simulink model "INS"  (R2018b)
settings: configuration reference "ins_config" (kept outside this file)
values from neighbouring files (symbols this model uses):
  INS_EXPORT = Simulink.Parameter(INS_EXPORT_VALUE)    [ins_model_init.m]
  INS_PARAM = Simulink.Parameter(INS_PARAM_VALUE)    [ins_model_init.m]
undefined symbols (not defined in the file or in its folder): DiscIntNeverNeededParam, INS_CONST, INS_EXPORT_VALUE
libraries: simulink x90, FMT_Model_Lib x31
(part 2 of 4)

== system INS/Bus_Constructor/Status_Output/INS_Flag/valid_check8 ==
  quality : Inport
  Compare To Constant : simulink/Logic and Bit Operations/Compare To Constant  relop=>=  const=time_out  OutDataTypeStr=boolean
  Compare To Constant1 : simulink/Logic and Bit Operations/Compare To Constant  relop=>  const=0  OutDataTypeStr=boolean
  Compare To Constant2 : simulink/Logic and Bit Operations/Compare To Constant  relop=>  const=0  OutDataTypeStr=boolean
  Constant : Constant  Value=INS_EXPORT.period  OutDataTypeStr=Inherit: Inherit via back propagation
  Delay : Delay  DelayLength=1
  Detect Rise Positive : simulink/Logic and Bit Operations/Detect Rise Positive  vinit=0  OutDataTypeStr=boolean
  Discrete-Time Integrator : DiscreteIntegrator  IntegratorMethod=Accumulation: Forward Euler  gainval=1  ExternalReset=level  SampleTime=-1  LimitOutput=on  UpperSaturationLimit=1e6  LowerSaturationLimit=0  ICPrevOutput=DiscIntNeverNeededParam  ICPrevScaledInput=DiscIntNeverNeededParam
  Logical Operator : Logic  Operator=NOT  AllPortsSameDT=off  OutDataTypeStr=boolean
  Logical Operator1 : Logic  Operator=OR  AllPortsSameDT=off  OutDataTypeStr=boolean
  Multiply : Product
  valid : Outport
  wires:
  Multiply/1 -> valid/1
  Delay/1 -> Multiply/2, Logical Operator1/2
  Logical Operator1/1 -> Delay/1
  Detect Rise Positive/1 -> Logical Operator1/1
  Compare To Constant2/1 -> Detect Rise Positive/1
  quality/1 -> Compare To Constant1/1, Compare To Constant2/1
  Compare To Constant1/1 -> Discrete-Time Integrator/2
  Constant/1 -> Discrete-Time Integrator/1
  Discrete-Time Integrator/1 -> Compare To Constant/1
  Compare To Constant/1 -> Logical Operator/1
  Logical Operator/1 -> Multiply/1

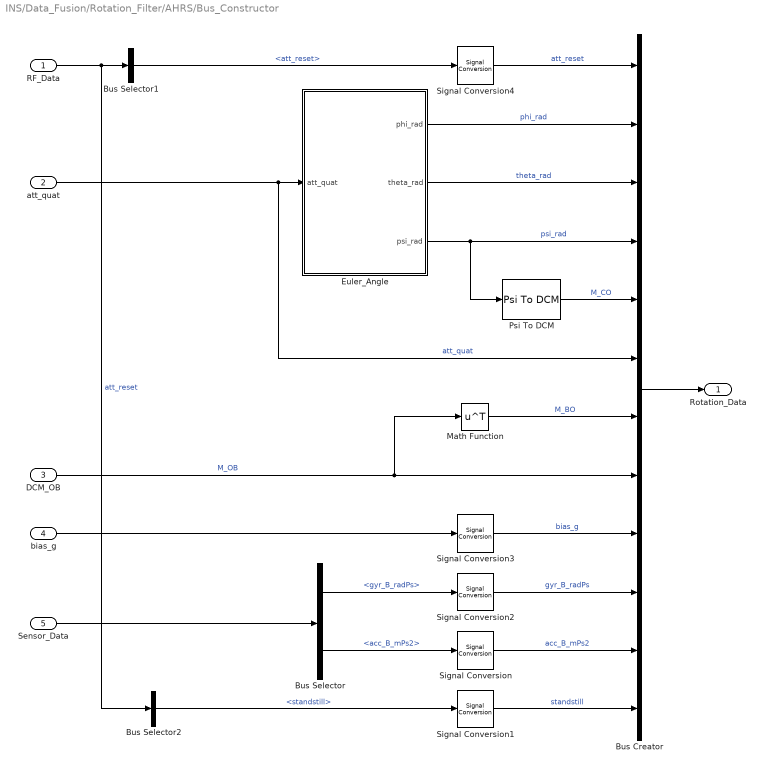
== system INS/Data_Fusion/Rotation_Filter/AHRS/Bus_Constructor ==
  RF_Data : Inport
  att_quat : Inport  Port=2
  DCM_OB : Inport  Port=3
  bias_g : Inport  Port=4
  Sensor_Data : Inport  Port=5
  Bus Creator : BusCreator  Inputs=12
  Bus Selector : BusSelector  OutputSignals=IMU_Data.gyr_B_radPs,IMU_Data.acc_B_mPs2
  Bus Selector1 : BusSelector  OutputSignals=att_reset
  Bus Selector2 : BusSelector  OutputSignals=standstill
  Euler_Angle : Subsystem
  Math Function : Math  Operator=transpose  SaturateOnIntegerOverflow=on
  Psi To DCM : FMT_Model_Lib/Transformation/Psi To DCM
      settings: SourceProductName=FMT Toolbox
  Signal Conversion{,1..4} (5 alike) : SignalConversion  OverrideOpt=off
  Rotation_Data : Outport
  wires:
  Bus Selector1/1 -> Signal Conversion4/1  "<att_reset>"
  Signal Conversion/1 -> Bus Creator/11  "acc_B_mPs2"
  Euler_Angle/1(phi_rad) -> Bus Creator/2  "phi_rad"
  Euler_Angle/2(theta_rad) -> Bus Creator/3  "theta_rad"
  Euler_Angle/3(psi_rad) -> Psi To DCM/1, Bus Creator/4  "psi_rad"
  Sensor_Data/1 -> Bus Selector/1
  Bus Selector2/1 -> Signal Conversion1/1  "<standstill>"
  Bus Creator/1 -> Rotation_Data/1
  bias_g/1 -> Signal Conversion3/1
  Math Function/1 -> Bus Creator/7  "M_BO"
  DCM_OB/1 -> Math Function/1, Bus Creator/8  "M_OB"
  att_quat/1 -> Euler_Angle/1(att_quat), Bus Creator/6  "att_quat"
  Psi To DCM/1 -> Bus Creator/5  "M_CO"
  Signal Conversion1/1 -> Bus Creator/12  "standstill"
  Bus Selector/2 -> Signal Conversion/1  "<acc_B_mPs2>"
  Signal Conversion2/1 -> Bus Creator/10  "gyr_B_radPs"
  Signal Conversion3/1 -> Bus Creator/9  "bias_g"
  RF_Data/1 -> Bus Selector2/1, Bus Selector1/1  "att_reset"
  Bus Selector/1 -> Signal Conversion2/1  "<gyr_B_radPs>"
  Signal Conversion4/1 -> Bus Creator/1  "att_reset"

== system INS/Data_Fusion/Rotation_Filter/AHRS/Correct ==
  Rotation_Data : Inport
  Sensor_Data : Inport  Port=2
  RF_Data : Inport  Port=3
  Attitude_Correction : Subsystem
  Bus Selector : BusSelector  OutputSignals=standstill
  Bus Selector1 : BusSelector  OutputSignals=IMU_Data
  Gyro_Bias_Correction : Subsystem
  att_B_correction : Outport
  bias_g_B_correction : Outport  Port=2
  wires:
  Gyro_Bias_Correction/1(bias_g_B_correction) -> bias_g_B_correction/1
  Bus Selector1/1 -> Gyro_Bias_Correction/2(IMU_Data)  "<IMU_Data>"
  RF_Data/1 -> Bus Selector/1
  Attitude_Correction/1(att_B_correction) -> att_B_correction/1, Gyro_Bias_Correction/1(att_B_correction)
  Sensor_Data/1 -> Attitude_Correction/1(Sensor_Data), Bus Selector1/1
  Rotation_Data/1 -> Attitude_Correction/2(Rotation_Data)
  Bus Selector/1 -> Attitude_Correction/3(standstill)  "<standstill>"

== system INS/Data_Fusion/Rotation_Filter/AHRS/Update ==
  att_B_correction : Inport
  bias_g_correction : Inport  Port=2
  RF_Data : Inport  Port=3
  Sensor_Data : Inport  Port=4
  Attitude_Update : Subsystem
  Bus Selector : BusSelector  OutputSignals=IMU_Data.gyr_B_radPs
  Bus Selector1 : BusSelector  OutputSignals=att_reset,quat_0
  Gyro_Bias_Update : Subsystem
  Sum2 : Sum  Inputs=|++
  att_quat : Outport
  DCM_OB : Outport  Port=2
  bias_g : Outport  Port=3
  wires:
  Sensor_Data/1 -> Bus Selector/1
  Gyro_Bias_Update/1(gyr_B_correction) -> Sum2/2
  att_B_correction/1 -> Sum2/1
  Sum2/1 -> Attitude_Update/3(att_B_correction)
  Bus Selector/1 -> Gyro_Bias_Update/2(gyr_B_radPs)  "<gyr_B_radPs>"
  bias_g_correction/1 -> Gyro_Bias_Update/1(bias_g_correction)
  Attitude_Update/1(att_quat) -> att_quat/1
  Attitude_Update/2(DCM_OB) -> DCM_OB/1
  Gyro_Bias_Update/2(bias_g) -> bias_g/1
  RF_Data/1 -> Bus Selector1/1  "att_reset"
  Bus Selector1/1 -> Attitude_Update/1(att_reset)  "<att_reset>"
  Bus Selector1/2 -> Attitude_Update/2(quat_0)  "<quat_0>"

== system INS/Data_Fusion/Rotation_Filter/RF_Data_PreProcess/Attitude_Reset ==
  Sensor_Data : Inport
  Bus Selector : BusSelector  OutputSignals=IMU_Data.IMU_valid,Mag_Data.mag_quality,IMU_Data.acc_B_mPs2,Mag_Data.mag_norm_B
  Bus Selector1 : BusSelector  OutputSignals=GPS_Data.GPS_valid
  Compare To Constant : simulink/Logic and Bit Operations/Compare To Constant  relop=>  const=0.01  OutDataTypeStr=boolean
  Compare To Constant1 : simulink/Logic and Bit Operations/Compare To Constant  relop=>=  const=0.2  OutDataTypeStr=boolean
  Detect Rise Positive : simulink/Logic and Bit Operations/Detect Rise Positive  vinit=0  OutDataTypeStr=boolean
  Interval Test : simulink/Logic and Bit Operations/Interval Test  IntervalClosedRight=on  uplimit=INS_CONST.g+0.5  IntervalClosedLeft=on  lowlimit=INS_CONST.g-0.5  OutDataTypeStr=boolean
  Logical Operator : Logic  AllPortsSameDT=off  OutDataTypeStr=boolean
  Logical Operator1 : Logic  Inputs=4  AllPortsSameDT=off  OutDataTypeStr=boolean
  Logical Operator2 : Logic  Operator=OR  AllPortsSameDT=off  OutDataTypeStr=boolean
  Reset Heading : Subsystem
  Vector Modulus : FMT_Model_Lib/Math/Vector Modulus
      settings: SourceProductName=FMT Toolbox
  Vector Modulus1 : FMT_Model_Lib/Math/Vector Modulus
      settings: SourceProductName=FMT Toolbox
  sample_valid : Subsystem
  att_reset : Outport
  wires:
  sample_valid/1(sample_valid) -> Logical Operator/1, Detect Rise Positive/1
  Vector Modulus1/1 -> Compare To Constant/1
  Compare To Constant/1 -> Logical Operator1/4
  Interval Test/1 -> Logical Operator1/3
  Vector Modulus/1 -> Interval Test/1
  Logical Operator1/1 -> sample_valid/1(valid)
  Sensor_Data/1 -> Bus Selector1/1, Bus Selector/1
  Bus Selector/2 -> Compare To Constant1/1  "<mag_quality>"
  Bus Selector/3 -> Vector Modulus/1  "<acc_B_mPs2>"
  Bus Selector/1 -> Logical Operator1/1  "<IMU_valid>"
  Compare To Constant1/1 -> Logical Operator1/2
  Bus Selector/4 -> Vector Modulus1/1  "<mag_norm_B>"
  Detect Rise Positive/1 -> Logical Operator2/1
  Logical Operator/1 -> Logical Operator2/2
  Logical Operator2/1 -> att_reset/1
  Bus Selector1/1 -> Reset Heading/1(GPS_valid)  "<GPS_valid>"
  Reset Heading/1(reset) -> Logical Operator/2

== system INS/Data_Fusion/Rotation_Filter/RF_Data_PreProcess/Initial_Attitude ==
  Sensor_Data : Inport
  Enable : EnablePort
  Bus Selector : BusSelector  OutputSignals=IMU_Data.acc_B_mPs2,Mag_Data.mag_norm_B
  Cross Product : FMT_Model_Lib/Math/Cross Product
      settings: SourceProductName=FMT Toolbox
  Cross Product1 : FMT_Model_Lib/Math/Cross Product
      settings: SourceProductName=FMT Toolbox
  DCM To Quaternion : FMT_Model_Lib/Quaternion/DCM To Quaternion
      settings: SourceProductName=FMT Toolbox
  Gain : Gain  Gain=-1
  Vector Concatenate : Concatenate  NumInputs=3  Mode=Multidimensional array  ConcatenateDimension=2
  Vector Normalize : FMT_Model_Lib/Math/Vector Normalize
      settings: SourceProductName=FMT Toolbox
  Vector Normalize1 : FMT_Model_Lib/Math/Vector Normalize
      settings: SourceProductName=FMT Toolbox
  Vector Normalize2 : FMT_Model_Lib/Math/Vector Normalize
      settings: SourceProductName=FMT Toolbox
  quat_0 : Outport  InitialOutput=[1; 0; 0; 0]
  wires:
  Gain/1 -> Cross Product/1, Vector Normalize2/1, Cross Product1/2
  Cross Product1/1 -> Vector Normalize/1
  Cross Product/1 -> Vector Normalize1/1, Cross Product1/1
  Vector Normalize1/1 -> Vector Concatenate/2  "DCM_y"
  Vector Normalize/1 -> Vector Concatenate/1  "DCM_x"
  Vector Normalize2/1 -> Vector Concatenate/3  "DCM_z"
  DCM To Quaternion/1 -> quat_0/1
  Sensor_Data/1 -> Bus Selector/1
  Bus Selector/1 -> Gain/1  "<acc_B_mPs2>"
  Bus Selector/2 -> Cross Product/2  "<mag_norm_B>"
  Vector Concatenate/1 -> DCM To Quaternion/1  "M_BO"

== system INS/Data_Fusion/Rotation_Filter/RF_Data_PreProcess/Standstill ==
  IMU_Data : Inport
  Abs : Abs
  Bus Selector : BusSelector  OutputSignals=gyr_B_radPs
  First Order HPF : FMT_Model_Lib/Filter/First Order HPF  fc=1/(2*pi*0.25)
      settings: SourceProductName=FMT Toolbox
  First Order LPF : FMT_Model_Lib/Filter/First Order LPF  fc=1/(2*pi*0.5)
      settings: SourceProductName=FMT Toolbox
  First Order LPF1 : FMT_Model_Lib/Filter/First Order LPF  fc=1/(2*pi*0.05)
      settings: SourceProductName=FMT Toolbox
  MinMax1 : MinMax  Function=max
  Relay : Relay  OnSwitchValue=10e-3  OffSwitchValue=3e-3  OnOutputValue=0  OffOutputValue=1
  Saturation2 : Saturate  UpperLimit=1  LowerLimit=0
  Selector : Selector  InputPortWidth=3  IndexOptions=Index vector (dialog)  Indices=[1 2]  OutputSizes=1
  standstill : Outport
  wires:
  First Order LPF1/1 -> Relay/1
  Relay/1 -> standstill/1
  Saturation2/1 -> First Order LPF1/1
  First Order HPF/1 -> Abs/1
  Selector/1 -> First Order HPF/1
  Abs/1 -> MinMax1/1
  First Order LPF/1 -> Saturation2/1
  MinMax1/1 -> First Order LPF/1
  Bus Selector/1 -> Selector/1  "<gyr_B_radPs>"
  IMU_Data/1 -> Bus Selector/1

== system INS/Data_Fusion/Translation_Filter/CF/Bus_Constructor ==
  TF_Data : Inport
  Horizontal_States : Inport  Port=2
  Verticle_States : Inport  Port=3
  Bus Creator : BusCreator  Inputs=16
  Bus Selector : BusSelector  OutputSignals=Sensor_Enable,TF_Control.WGS84_Ref.WGS84_pos_ref.lat_0_rad,TF_Control.WGS84_Ref.WGS84_pos_ref.lon_0_rad,TF_Control.WGS84_Ref.WGS84_pos_ref.h_0_m
  Bus_Select : Subsystem
  Constant : Constant  OutDataTypeStr=Inherit: Inherit via back propagation
  Signal Copy{,1..3} (4 alike) : SignalConversion  OverrideOpt=off
  Translation_Data : Outport
  wires:
  Bus Creator/1 -> Translation_Data/1
  Bus_Select/10(vd_mPs) -> Bus Creator/10  "vd_mPs"
  Bus_Select/9(ve_mPs) -> Bus Creator/9  "ve_mPs"
  Bus_Select/8(vn_mPs) -> Bus Creator/8  "vn_mPs"
  Bus_Select/3(h_m) -> Bus Creator/3  "h_m"
  Bus_Select/2(lon_rad) -> Bus Creator/2  "lon_rad"
  Bus_Select/1(lat_rad) -> Bus Creator/1  "lat_rad"
  Bus_Select/11(ba_mPs2) -> Bus Creator/11  "ba_mPs2"
  Verticle_States/1 -> Bus_Select/2(Verticle_States)
  Horizontal_States/1 -> Bus_Select/1(Horizontal_States)
  TF_Data/1 -> Bus Selector/1, Bus_Select/3(TF_Data)
  Constant/1 -> Bus Creator/16  "init_done"
  Bus_Select/7(h_gnd_m) -> Bus Creator/7  "h_gnd_m"
  Bus_Select/6(h_R_m) -> Bus Creator/6  "h_R_m"
  Bus_Select/4(x_R_m) -> Bus Creator/4  "x_R_m"
  Bus_Select/5(y_R_m) -> Bus Creator/5  "y_R_m"
  Bus Selector/1 -> Signal Copy/1  "<Sensor_Enable>"
  Signal Copy/1 -> Bus Creator/12  "sensor_enable"
  Bus Selector/2 -> Signal Copy1/1  "<lat_0_rad>"
  Bus Selector/3 -> Signal Copy2/1  "<lon_0_rad>"
  Bus Selector/4 -> Signal Copy3/1  "<h_0_m>"
  Signal Copy1/1 -> Bus Creator/13  "lat_0_rad"
  Signal Copy2/1 -> Bus Creator/14  "lon_0_rad"
  Signal Copy3/1 -> Bus Creator/15  "h_0_m"

== system INS/Data_Fusion/Translation_Filter/CF/Horizontal_Filter ==
  TF_Data : Inport
  Rotation_Data : Inport  Port=2
  Correct : Subsystem
  Predict : Subsystem
  Reshape : Reshape  OutputDimensionality=Customize  OutputDimensions=[6,1]
  States : Outport
  wires:
  Predict/1(X_Predict) -> Correct/1(X_Predict)
  Correct/1(X_Next) -> Reshape/1
  Reshape/1 -> Predict/1(X_Prio), States/1
  TF_Data/1 -> Correct/2(TF_Data), Predict/3(TF_Data)
  Rotation_Data/1 -> Predict/2(Rotation_Data)

== system INS/Data_Fusion/Translation_Filter/CF/Verticle_Filter ==
  TF_Data : Inport
  Rotation_Data : Inport  Port=2
  Correct : Subsystem
  Predict : Subsystem
  Reshape : Reshape  OutputDimensionality=Customize  OutputDimensions=[3,1]
  States : Outport
  wires:
  Predict/1(X_Predict) -> Correct/1(X_Predict)
  Correct/1(X_Next) -> Reshape/1
  Reshape/1 -> Predict/1(X_Prio), States/1
  TF_Data/1 -> Correct/2(TF_Data), Predict/3(TF_Data)
  Rotation_Data/1 -> Predict/2(Rotation_Data)

== system INS/Data_Fusion/Translation_Filter/TF_Data_PreProcess/Sensor_Process ==
  Sensor_Data : Inport
  Sensor_Select : Subsystem
  TF_Sensor_Measures : Subsystem
  TF_Sensor_Status : Subsystem
  Sensor_Status : Outport
  Sensor_Meas : Outport  Port=2
  Sensor_Enable : Outport  Port=3
  wires:
  Sensor_Data/1 -> TF_Sensor_Measures/1(Sensor_Data), TF_Sensor_Status/1(Sensor_Data)
  TF_Sensor_Measures/1(Sensor_Meas) -> Sensor_Meas/1
  TF_Sensor_Status/1(Sensor_Status) -> Sensor_Select/1(Sensor_Status), Sensor_Status/1
  Sensor_Select/1(Sensor_Select) -> Sensor_Enable/1  "Sensor_Enable"

== system INS/Data_Fusion/Translation_Filter/TF_Data_PreProcess/Transfer_Filter_Control ==
  Sensor_Enable : Inport
  Sensor_Meas : Inport  Port=2
  Translation_Data : Inport  Port=3
  Bus Creator : BusCreator  Inputs=4
  Filter_Reset : Subsystem
  Position_Reference : Subsystem
  Sensor_Valid : Subsystem
  TF_Control : Outport
  wires:
  Position_Reference/1(WGS84_Ref) -> Bus Creator/4  "WGS84_Ref"
  Sensor_Meas/1 -> Position_Reference/3(Sensor_Meas)
  Filter_Reset/1(pos_reset) -> Bus Creator/1  "pos_reset"
  Sensor_Enable/1 -> Sensor_Valid/1(Sensor_Enable)
  Filter_Reset/2(height_reset) -> Bus Creator/2  "height_reset"
  Bus Creator/1 -> TF_Control/1
  Translation_Data/1 -> Position_Reference/2(Translation_Data)
  Sensor_Valid/1(Sensor_Valid) -> Position_Reference/1(Sensor_Valid), Bus Creator/3, Filter_Reset/1(Sensor_Valid)  "sensor_valid"

== system INS/Sensor_PreProcess/Baro_Process/Relative_Height/Reference_Height ==
  h_FL_m : Inport
  Enable : EnablePort  StatesWhenEnabling=reset
  Constant1 : Constant  OutDataTypeStr=uint32
  Delay : Delay  DelayLength=1
  Delay1 : Delay  DelayLength=1
  Divide : Product  Inputs=*/
  Saturation1 : Saturate  UpperLimit=10000  LowerLimit=1
  Sum1 : Sum  Inputs=|++  AccumDataTypeStr=uint32  OutDataTypeStr=uint32  RndMeth=Simplest  SaturateOnIntegerOverflow=on
  Sum2 : Sum  Inputs=|++
  h_R_m : Outport
  wires:
  Saturation1/1 -> Divide/2
  Constant1/1 -> Sum1/1
  Sum1/1 -> Delay1/1, Saturation1/1
  Delay1/1 -> Sum1/2
  Sum2/1 -> Delay/1, Divide/1
  Delay/1 -> Sum2/2
  h_FL_m/1 -> Sum2/1
  Divide/1 -> h_R_m/1

== system INS/Sensor_PreProcess/Baro_Process/Relative_Height/Sampling ==
  timestamp : Inport
  data_valid : Inport  Port=2
  Compare To Constant : simulink/Logic and Bit Operations/Compare To Constant  relop=>  const=200  OutDataTypeStr=boolean
  Delay : Delay  DelayLength=1
  Detect Change : simulink/Logic and Bit Operations/Detect Change  vinit=0  OutDataTypeStr=boolean
  Interval Test3 : simulink/Logic and Bit Operations/Interval Test  IntervalClosedRight=off  uplimit=200  IntervalClosedLeft=off  lowlimit=1  OutDataTypeStr=boolean
  Logical Operator5 : Logic  AllPortsSameDT=off  OutDataTypeStr=boolean
  Saturation : Saturate  UpperLimit=10000  LowerLimit=0
  Sum1 : Sum  Inputs=|++  AccumDataTypeStr=uint32  OutDataTypeStr=uint32  RndMeth=Simplest  SaturateOnIntegerOverflow=on
  sampling : Outport
  initialized : Outport  Port=2
  wires:
  Detect Change/1 -> Logical Operator5/1
  Interval Test3/1 -> sampling/1
  Logical Operator5/1 -> Sum1/1
  Delay/1 -> Saturation/1
  timestamp/1 -> Detect Change/1
  data_valid/1 -> Logical Operator5/2
  Sum1/1 -> Interval Test3/1, Compare To Constant/1, Delay/1
  Saturation/1 -> Sum1/2
  Compare To Constant/1 -> initialized/1

== system INS/Sensor_PreProcess/GPS_PreProcess/Status_Quality/GPS_Status ==
  note: GPS Status
      | 0: Idle
      | 1: Ready, 3D fix lost
      | 2: Ready, 3D fix
  not_timeout : Inport
  hAcc : Inport  Port=2
  fixtype : Inport  Port=3
  Compare To Constant : simulink/Logic and Bit Operations/Compare To Constant  relop=<  const=5*1e3  OutDataTypeStr=uint8
  Compare To Constant1 : simulink/Logic and Bit Operations/Compare To Constant  relop===  const=3  OutDataTypeStr=uint8
  Logical Operator : Logic  Inputs=3  AllPortsSameDT=off  OutDataTypeStr=fixdt(0,8)
  Logical Operator1 : Logic  Inputs=3  AllPortsSameDT=off  OutDataTypeStr=fixdt(0,8)
  Ready : Subsystem
  Sum1 : Sum  Inputs=|++
  status : Outport
  wires:
  not_timeout/1 -> Logical Operator/3, Logical Operator1/3
  Sum1/1 -> status/1
  Logical Operator1/1 -> Sum1/2  "3D Fix"
  hAcc/1 -> Compare To Constant/1
  Compare To Constant/1 -> Logical Operator/1
  Compare To Constant1/1 -> Logical Operator1/2, Logical Operator/2  "3D Fix"
  fixtype/1 -> Compare To Constant1/1
  Ready/1(ready) -> Sum1/1, Logical Operator1/1  "ready"
  Logical Operator/1 -> Ready/1(valid)

== system INS/Sensor_PreProcess/GPS_PreProcess/Status_Quality/check_timeout ==
  timestamp : Inport
  Compare To Constant4 : simulink/Logic and Bit Operations/Compare To Constant  relop=<  const=500  OutDataTypeStr=boolean
  Constant : Constant  Value=INS_EXPORT.period  OutDataTypeStr=single
  Detect Change : simulink/Logic and Bit Operations/Detect Change  vinit=0  OutDataTypeStr=boolean
  Discrete-Time Integrator : DiscreteIntegrator  IntegratorMethod=Accumulation: Forward Euler  ExternalReset=sampled level  SampleTime=-1  OutDataTypeStr=uint32  SaturateOnIntegerOverflow=on  UpperSaturationLimit=10000  LowerSaturationLimit=0  ICPrevOutput=DiscIntNeverNeededParam  ICPrevScaledInput=DiscIntNeverNeededParam
  valid : Outport
  wires:
  Constant/1 -> Discrete-Time Integrator/1
  timestamp/1 -> Detect Change/1
  Detect Change/1 -> Discrete-Time Integrator/2
  Discrete-Time Integrator/1 -> Compare To Constant4/1
  Compare To Constant4/1 -> valid/1

== system INS/Sensor_PreProcess/GPS_PreProcess/Status_Quality/horizontal_quality ==
  hAcc : Inport
  Constant1 : Constant  Value=INS_PARAM.GPS_HOR_Q_BIAS  OutDataTypeStr=Inherit: Inherit via back propagation
  Gain1 : Gain  Gain=1e-3  OutDataTypeStr=single
  Gain2 : Gain  Gain=INS_PARAM.GPS_HOR_Q_SCALE  OutDataTypeStr=single
  Saturation1 : Saturate  UpperLimit=1  LowerLimit=0
  Sum1 : Sum  Inputs=+-|
  hor_quality : Outport
  wires:
  Sum1/1 -> Gain2/1
  Gain1/1 -> Sum1/2  "hAcc_m"
  hAcc/1 -> Gain1/1
  Constant1/1 -> Sum1/1
  Gain2/1 -> Saturation1/1
  Saturation1/1 -> hor_quality/1

== system INS/Sensor_PreProcess/GPS_PreProcess/Status_Quality/speed_acc ==
  sAcc : Inport
  Constant7 : Constant  Value=INS_PARAM.GPS_VEL_Q_BIAS  OutDataTypeStr=Inherit: Inherit via back propagation
  Gain3 : Gain  Gain=INS_PARAM.GPS_VEL_Q_SCALE  OutDataTypeStr=single
  Gain5 : Gain  Gain=1e-3  OutDataTypeStr=single
  Saturation : Saturate  UpperLimit=1  LowerLimit=0
  Second Order LPF : FMT_Model_Lib/Filter/Second Order LPF  fc=5  zeta=0.707
      settings: SourceProductName=FMT Toolbox
  Sum : Sum  Inputs=+-|
  spd_quality : Outport
  wires:
  Gain5/1 -> Sum/2  "sAcc_m"
  Sum/1 -> Gain3/1
  sAcc/1 -> Gain5/1
  Constant7/1 -> Sum/1
  Saturation/1 -> spd_quality/1
  Gain3/1 -> Second Order LPF/1
  Second Order LPF/1 -> Saturation/1

== system INS/Sensor_PreProcess/GPS_PreProcess/Status_Quality/vertical_quality ==
  vAcc : Inport
  Constant1 : Constant  Value=INS_PARAM.GPS_VER_Q_BIAS  OutDataTypeStr=Inherit: Inherit via back propagation
  Gain1 : Gain  Gain=1e-3  OutDataTypeStr=single
  Gain2 : Gain  Gain=INS_PARAM.GPS_VER_Q_SCALE  OutDataTypeStr=single
  Saturation1 : Saturate  UpperLimit=1  LowerLimit=0
  Sum1 : Sum  Inputs=+-|
  ver_quality : Outport
  wires:
  Sum1/1 -> Gain2/1
  Gain1/1 -> Sum1/2  "vAcc_m"
  vAcc/1 -> Gain1/1
  Constant1/1 -> Sum1/1
  Gain2/1 -> Saturation1/1
  Saturation1/1 -> ver_quality/1

== system INS/Sensor_PreProcess/MAG_PreProcess/Mag_Data_Process/Mag_Quality_Estimate ==
  note: TODO: improve this
  mag_normalized_O : Inport
  nominal_inc_deg : Inport  Port=2
  pos_0_valid : Inport  Port=3
  mag_valid : Inport  Port=4
  Mag_Quality : Subsystem
  Multiply : Product  OutDataTypeStr=Inherit: Same as first input
  Switch : Switch  Criteria=u2 > Threshold
  default_mag_quality : Constant  Value=0.5  OutDataTypeStr=single
  mag_quality : Outport
  wires:
  pos_0_valid/1 -> Switch/2
  default_mag_quality/1 -> Switch/3
  mag_valid/1 -> Multiply/2
  Switch/1 -> Multiply/1
  Multiply/1 -> mag_quality/1
  nominal_inc_deg/1 -> Mag_Quality/1(nominal_inc_deg)
  mag_normalized_O/1 -> Mag_Quality/2(mag_normalized_O)
  Mag_Quality/1(mag_quality) -> Switch/1

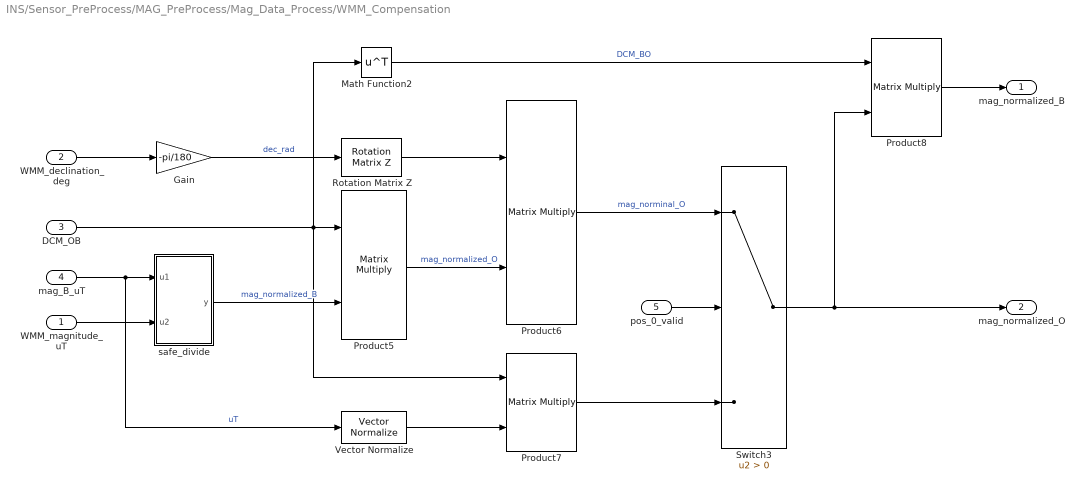
== system INS/Sensor_PreProcess/MAG_PreProcess/Mag_Data_Process/WMM_Compensation ==
  WMM_magnitude_uT : Inport
  WMM_declination_deg : Inport  Port=2
  DCM_OB : Inport  Port=3
  mag_B_uT : Inport  Port=4
  pos_0_valid : Inport  Port=5
  Gain : Gain  Gain=-pi/180  OutDataTypeStr=single
  Math Function2 : Math  Operator=transpose  SaturateOnIntegerOverflow=on
  Product{5..8} (4 alike) : Product  Multiplication=Matrix(*)
  Rotation Matrix Z : FMT_Model_Lib/Transformation/Rotation Matrix Z
      settings: SourceProductName=FMT Toolbox
  Switch3 : Switch  Criteria=u2 > Threshold
  Vector Normalize : FMT_Model_Lib/Math/Vector Normalize
      settings: SourceProductName=FMT Toolbox
  safe_divide : Subsystem
      mask Display:
      | port_label('input', 1, 'x', 'texmode', 'on')
      | port_label('input', 2, '÷', 'texmode', 'on')
  mag_normalized_B : Outport
  mag_normalized_O : Outport  Port=2
  wires:
  Gain/1 -> Rotation Matrix Z/1  "dec_rad"
  WMM_declination_deg/1 -> Gain/1
  mag_B_uT/1 -> Vector Normalize/1, safe_divide/1(u1)  "uT"
  WMM_magnitude_uT/1 -> safe_divide/2(u2)
  safe_divide/1(y) -> Product5/2  "mag_normalized_B"
  DCM_OB/1 -> Product5/1, Math Function2/1, Product7/1
  Product5/1 -> Product6/2  "mag_normalized_O"
  Rotation Matrix Z/1 -> Product6/1
  Product6/1 -> Switch3/1  "mag_norminal_O"
  Math Function2/1 -> Product8/1  "DCM_BO"
  pos_0_valid/1 -> Switch3/2
  Product8/1 -> mag_normalized_B/1
  Switch3/1 -> mag_normalized_O/1, Product8/2
  Vector Normalize/1 -> Product7/2
  Product7/1 -> Switch3/3

== system INS/Sensor_PreProcess/MAG_PreProcess/Mag_Data_Process/WMM_LUT ==
  lat_rad : Inport
  lon_rad : Inport  Port=2
  Add : Sum
  Declination_Lookup_Table : LookupNDDirect  Table=wmm_declination  DiagnosticForOutOfRangeInput=Error
  Demux : Demux  Outputs=2
  Inclination_Lookup_Table : LookupNDDirect  Table=wmm_inclination  DiagnosticForOutOfRangeInput=Error
  Magnitude_Lookup_Table : LookupNDDirect  Table=wmm_magnitude  DiagnosticForOutOfRangeInput=Error
  Mux : Mux  Inputs=2
  Saturation1 : Saturate  UpperLimit=size(wmm_magnitude)-1  LowerLimit=0
  offset : Constant  Value=(size(wmm_magnitude)-1)/2  OutDataTypeStr=int32
  rad_to_index : Gain  Gain=180/pi/resolution  OutDataTypeStr=int32
  magnitude_uT : Outport
  declination_deg : Outport  Port=2
  inclination_deg : Outport  Port=3
  wires:
  Inclination_Lookup_Table/1 -> inclination_deg/1
  Declination_Lookup_Table/1 -> declination_deg/1
  Magnitude_Lookup_Table/1 -> magnitude_uT/1
  offset/1 -> Add/2
  Add/1 -> Saturation1/1
  rad_to_index/1 -> Add/1
  lat_rad/1 -> Mux/1
  lon_rad/1 -> Mux/2
  Mux/1 -> rad_to_index/1
  Saturation1/1 -> Demux/1
  Demux/1 -> Magnitude_Lookup_Table/1, Inclination_Lookup_Table/1, Declination_Lookup_Table/1
  Demux/2 -> Inclination_Lookup_Table/2, Magnitude_Lookup_Table/2, Declination_Lookup_Table/2

== system INS/Data_Fusion/Rotation_Filter/AHRS/Bus_Constructor/Euler_Angle ==
  att_quat : Inport
  Demux : Demux  Outputs=3
  Quaternion To Euler : FMT_Model_Lib/Quaternion/Quaternion To Euler
      settings: SourceProductName=FMT Toolbox
  phi_rad : Outport
  theta_rad : Outport  Port=2
  psi_rad : Outport  Port=3
  wires:
  Demux/1 -> phi_rad/1
  Demux/2 -> theta_rad/1
  Demux/3 -> psi_rad/1
  att_quat/1 -> Quaternion To Euler/1
  Quaternion To Euler/1 -> Demux/1

== system INS/Data_Fusion/Rotation_Filter/AHRS/Correct/Attitude_Correction ==
  Sensor_Data : Inport
  Rotation_Data : Inport  Port=2
  standstill : Inport  Port=3
  Attitude_Correct : Subsystem
  Bus Selector2 : BusSelector  OutputSignals=M_BO
  Mag_Correct : Subsystem
  Multiply : Product  Multiplication=Matrix(*)
  Sum : Sum  Inputs=|++
  att_B_correction : Outport
  wires:
  standstill/1 -> Mag_Correct/3(standstill)
  Sensor_Data/1 -> Attitude_Correct/2(Sensor_Data), Mag_Correct/2(Sensor_Data)
  Attitude_Correct/1(att_corr_O) -> Sum/1  "att_corr_O"
  Mag_Correct/1(mag_corr_O) -> Sum/2  "mag_corr_O"
  Multiply/1 -> att_B_correction/1
  Rotation_Data/1 -> Mag_Correct/1(Rotation_Data), Attitude_Correct/1(Rotation_Data), Bus Selector2/1
  Sum/1 -> Multiply/2
  Bus Selector2/1 -> Multiply/1  "<M_BO>"

== system INS/Data_Fusion/Rotation_Filter/AHRS/Correct/Gyro_Bias_Correction ==
  att_B_correction : Inport
  IMU_Data : Inport  Port=2
  Abs : Abs
  Bus Selector : BusSelector  OutputSignals=acc_B_mPs2
  Compare To Constant : simulink/Logic and Bit Operations/Compare To Constant  relop=<=  const=1  OutDataTypeStr=boolean
  Constant : Constant  Value=INS_CONST.g  OutDataTypeStr=single
  Data Type Conversion : DataTypeConversion  OutDataTypeStr=single
  Gain1 : Gain  Gain=INS_PARAM.BIAS_G_CORR_GAIN
  MX Product1 : Product  RndMeth=Simplest
  Saturation2 : Saturate  UpperLimit=0.1/180*pi  LowerLimit=-0.1/180*pi
  Second Order LPF : FMT_Model_Lib/Filter/Second Order LPF  fc=5  zeta=0.707
      settings: SourceProductName=FMT Toolbox
  Subtract : Sum  Inputs=+-
  Vector Modulus : FMT_Model_Lib/Math/Vector Modulus
      settings: SourceProductName=FMT Toolbox
  bias_g_B_correction : Outport
  wires:
  IMU_Data/1 -> Bus Selector/1
  Saturation2/1 -> bias_g_B_correction/1  "bias_g_correction"
  Compare To Constant/1 -> Data Type Conversion/1
  Bus Selector/1 -> Vector Modulus/1  "<acc_B_mPs2>"
  MX Product1/1 -> Second Order LPF/1
  att_B_correction/1 -> MX Product1/1
  Vector Modulus/1 -> Subtract/1
  Gain1/1 -> Saturation2/1
  Constant/1 -> Subtract/2
  Subtract/1 -> Abs/1
  Abs/1 -> Compare To Constant/1
  Data Type Conversion/1 -> MX Product1/2
  Second Order LPF/1 -> Gain1/1

== system INS/Data_Fusion/Rotation_Filter/AHRS/Update/Attitude_Update ==
  att_reset : Inport
  quat_0 : Inport  Port=2
  att_B_correction : Inport  Port=3
  Constant : Constant  Value=0  OutDataTypeStr=single
  Discrete-Time Integrator : DiscreteIntegrator  ExternalReset=level  InitialConditionSource=external  SampleTime=-1  ICPrevOutput=DiscIntNeverNeededParam  ICPrevScaledInput=DiscIntNeverNeededParam
  Gain2 : Gain  Gain=0.5  OutMin=-450*pi/180  OutMax=450*pi/180  RndMeth=Simplest
  Mux1 : Mux  Inputs=2
  Quaternion Multiply : FMT_Model_Lib/Quaternion/Quaternion Multiply
      settings: SourceProductName=FMT Toolbox
  Quaternion Normalize : FMT_Model_Lib/Quaternion/Quaternion Normalize
      settings: SourceProductName=FMT Toolbox
  Quaternion To DCM : FMT_Model_Lib/Quaternion/Quaternion To DCM
      settings: SourceProductName=FMT Toolbox
  Transpose : Math  Operator=transpose  SaturateOnIntegerOverflow=on
  att_quat : Outport
  DCM_OB : Outport  Port=2
  wires:
  att_reset/1 -> Discrete-Time Integrator/2
  quat_0/1 -> Discrete-Time Integrator/3
  Gain2/1 -> Discrete-Time Integrator/1
  Quaternion Multiply/1 -> Gain2/1
  att_B_correction/1 -> Mux1/2
  Mux1/1 -> Quaternion Multiply/2
  Constant/1 -> Mux1/1
  Quaternion Normalize/1 -> Quaternion To DCM/1, Quaternion Multiply/1, att_quat/1
  Discrete-Time Integrator/1 -> Quaternion Normalize/1
  Quaternion To DCM/1 -> Transpose/1
  Transpose/1 -> DCM_OB/1

== system INS/Data_Fusion/Rotation_Filter/AHRS/Update/Gyro_Bias_Update ==
  bias_g_correction : Inport
  gyr_B_radPs : Inport  Port=2
  Discrete-Time Integrator2 : DiscreteIntegrator  SampleTime=-1  LimitOutput=on  UpperSaturationLimit=45/180*pi  LowerSaturationLimit=-45/180*pi  ICPrevOutput=DiscIntNeverNeededParam  ICPrevScaledInput=DiscIntNeverNeededParam
  Sum1 : Sum  Inputs=++|
  gyr_B_correction : Outport
  bias_g : Outport  Port=2
  wires:
  bias_g_correction/1 -> Discrete-Time Integrator2/1
  Sum1/1 -> gyr_B_correction/1
  Discrete-Time Integrator2/1 -> Sum1/1, bias_g/1
  gyr_B_radPs/1 -> Sum1/2

== system INS/Data_Fusion/Rotation_Filter/RF_Data_PreProcess/Attitude_Reset/Reset Heading ==
  note: When GPS is valid at first time, the mag data will be compensated with WMM data,
      | so we need reset attitude.
  GPS_valid : Inport
  Add : Sum  AccumDataTypeStr=uint32
  Data Type Conversion : DataTypeConversion  OutDataTypeStr=uint32
  Delay : Delay  DelayLength=1
  Detect Rise Positive1 : simulink/Logic and Bit Operations/Detect Rise Positive  vinit=0  OutDataTypeStr=boolean
  Saturation : Saturate  UpperLimit=1  LowerLimit=0
  reset : Outport
  wires:
  Delay/1 -> Add/2
  Data Type Conversion/1 -> Add/1
  GPS_valid/1 -> Data Type Conversion/1
  Detect Rise Positive1/1 -> reset/1
  Add/1 -> Saturation/1
  Saturation/1 -> Detect Rise Positive1/1, Delay/1

== system INS/Data_Fusion/Rotation_Filter/RF_Data_PreProcess/Attitude_Reset/sample_valid ==
  valid : Inport
  Add : Sum  AccumDataTypeStr=uint32
  Data Type Conversion : DataTypeConversion  OutDataTypeStr=uint32
  Delay : Delay  DelayLength=1
  Saturation : Saturate  UpperLimit=10000  LowerLimit=0
  valid_samples : simulink/Logic and Bit Operations/Compare To Constant  relop=>  const=50  OutDataTypeStr=boolean
  sample_valid : Outport
  wires:
  Add/1 -> Saturation/1
  valid_samples/1 -> sample_valid/1
  Delay/1 -> Add/2
  valid/1 -> Data Type Conversion/1
  Data Type Conversion/1 -> Add/1
  Saturation/1 -> valid_samples/1, Delay/1

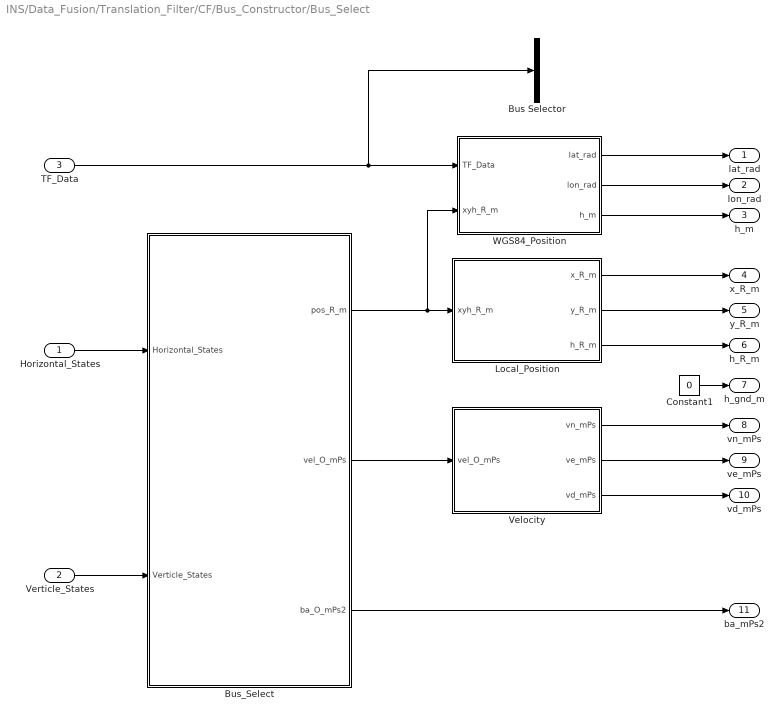
== system INS/Data_Fusion/Translation_Filter/CF/Bus_Constructor/Bus_Select ==
  Horizontal_States : Inport
  Verticle_States : Inport  Port=2
  TF_Data : Inport  Port=3
  Bus Selector : BusSelector  OutputSignals=TF_Control.WGS84_Ref.WGS84_pos_ref.lat_0_rad,TF_Control.WGS84_Ref.WGS84_pos_ref.lon_0_rad,TF_Control.WGS84_Ref.WGS84_pos_ref.h_0_m
  Bus_Select : Subsystem
  Constant1 : Constant  Value=0  OutDataTypeStr=Inherit: Inherit via back propagation
  Local_Position : Subsystem
  Velocity : Subsystem
  WGS84_Position : Subsystem
  lat_rad : Outport
  lon_rad : Outport  Port=2
  h_m : Outport  Port=3
  x_R_m : Outport  Port=4
  y_R_m : Outport  Port=5
  h_R_m : Outport  Port=6
  h_gnd_m : Outport  Port=7
  vn_mPs : Outport  Port=8
  ve_mPs : Outport  Port=9
  vd_mPs : Outport  Port=10
  ba_mPs2 : Outport  Port=11
  wires:
  WGS84_Position/1(lat_rad) -> lat_rad/1
  TF_Data/1 -> Bus Selector/1, WGS84_Position/1(TF_Data)
  WGS84_Position/2(lon_rad) -> lon_rad/1
  WGS84_Position/3(h_m) -> h_m/1
  Local_Position/1(x_R_m) -> x_R_m/1
  Local_Position/2(y_R_m) -> y_R_m/1
  Local_Position/3(h_R_m) -> h_R_m/1
  Bus_Select/1(pos_R_m) -> Local_Position/1(xyh_R_m), WGS84_Position/2(xyh_R_m)
  Horizontal_States/1 -> Bus_Select/1(Horizontal_States)
  Verticle_States/1 -> Bus_Select/2(Verticle_States)
  Bus_Select/3(ba_O_mPs2) -> ba_mPs2/1
  Constant1/1 -> h_gnd_m/1
  Bus_Select/2(vel_O_mPs) -> Velocity/1(vel_O_mPs)
  Velocity/1(vn_mPs) -> vn_mPs/1
  Velocity/2(ve_mPs) -> ve_mPs/1
  Velocity/3(vd_mPs) -> vd_mPs/1

== system INS/Data_Fusion/Translation_Filter/CF/Horizontal_Filter/Correct ==
  X_Predict : Inport
  TF_Data : Inport  Port=2
  Bus Selector : BusSelector  OutputSignals=Sensor_Enable.horizon_select.gps_enable
  GPS_Correct : Subsystem
  Switch : Switch  Criteria=u2 > Threshold
  X_Next : Outport
  wires:
  X_Predict/1 -> GPS_Correct/2(X_Predict), Switch/3
  TF_Data/1 -> GPS_Correct/1(TF_Data), Bus Selector/1
  Bus Selector/1 -> GPS_Correct/Enable, Switch/2  "<gps_enable>"
  Switch/1 -> X_Next/1
  GPS_Correct/1(X_Next) -> Switch/1

== system INS/Data_Fusion/Translation_Filter/CF/Horizontal_Filter/Predict ==
  X_Prio : Inport
  Rotation_Data : Inport  Port=2
  TF_Data : Inport  Port=3
  Propagate : Subsystem
  Update : Subsystem
  X_Predict : Outport
  wires:
  X_Prio/1 -> Propagate/1(X_prio)
  TF_Data/1 -> Propagate/2(TF_Data)
  Propagate/1(X) -> Update/1(X_Prio)
  Rotation_Data/1 -> Update/2(Rotation_Data)
  Update/1(X_Predict) -> X_Predict/1

== system INS/Data_Fusion/Translation_Filter/CF/Verticle_Filter/Correct ==
  X_Predict : Inport
  TF_Data : Inport  Port=2
  Baro_Correct : Subsystem
  GPS_Correct : Subsystem
  X_Next : Outport
  wires:
  TF_Data/1 -> GPS_Correct/2(TF_Data), Baro_Correct/2(TF_Data)
  X_Predict/1 -> Baro_Correct/1(X_Predict)
  Baro_Correct/1(X_Next) -> GPS_Correct/1(X_Predict)
  GPS_Correct/1(X_Next) -> X_Next/1

== system INS/Data_Fusion/Translation_Filter/CF/Verticle_Filter/Predict ==
  X_Prio : Inport
  Rotation_Data : Inport  Port=2
  TF_Data : Inport  Port=3
  Propagate : Subsystem
  Update : Subsystem
  X_Predict : Outport
  wires:
  X_Prio/1 -> Propagate/1(X_Prio)
  TF_Data/1 -> Propagate/2(TF_Data)
  Propagate/1(X) -> Update/1(X_Prio)
  Rotation_Data/1 -> Update/2(Rotation_Data)
  Update/1(X_Predict) -> X_Predict/1

== system INS/Data_Fusion/Translation_Filter/TF_Data_PreProcess/Sensor_Process/Sensor_Select ==
  Sensor_Status : Inport
  Bus Creator : BusCreator  Inputs=2
  Horizontal_Sensor_Select : Subsystem
  Vertical_Sensor_Select : Subsystem
  Sensor_Select : Outport
  wires:
  Sensor_Status/1 -> Vertical_Sensor_Select/1(Sensor_Status), Horizontal_Sensor_Select/1(Sensor_Status)
  Bus Creator/1 -> Sensor_Select/1
  Horizontal_Sensor_Select/1(horizon_select) -> Bus Creator/1  "horizon_select"
  Vertical_Sensor_Select/1(vert_select) -> Bus Creator/2  "vert_select"

== system INS/Data_Fusion/Translation_Filter/TF_Data_PreProcess/Sensor_Process/TF_Sensor_Measures ==
  Sensor_Data : Inport
  Barometer_Meas : Subsystem
  Bus Creator : BusCreator  Inputs=2
  GPS_Meas : Subsystem
  Sensor_Meas : Outport
  wires:
  Bus Creator/1 -> Sensor_Meas/1
  Sensor_Data/1 -> Barometer_Meas/1(Sensor_Data), GPS_Meas/1(Sensor_Data)
  GPS_Meas/1(GPS_Meas) -> Bus Creator/1  "GPS_Meas"
  Barometer_Meas/1(Baro_Meas) -> Bus Creator/2  "Baro_Meas"

== system INS/Data_Fusion/Translation_Filter/TF_Data_PreProcess/Sensor_Process/TF_Sensor_Status ==
  Sensor_Data : Inport
  Barometer_Status : Subsystem
  Bus Creator : BusCreator  Inputs=2
  GPS_Status : Subsystem
  Sensor_Status : Outport
  wires:
  Bus Creator/1 -> Sensor_Status/1
  Sensor_Data/1 -> Barometer_Status/1(Sensor_Data), GPS_Status/1(Sensor_Data)
  GPS_Status/1(GPS_Status) -> Bus Creator/1  "GPS_Status"
  Barometer_Status/1(Baro_Status) -> Bus Creator/2  "Baro_Status"

== system INS/Data_Fusion/Translation_Filter/TF_Data_PreProcess/Transfer_Filter_Control/Filter_Reset ==
  note: Height_Reset
  note: Position_Reset
  Sensor_Valid : Inport
  Bus Selector : BusSelector  OutputSignals=xy_R_valid
  Bus Selector1 : BusSelector  OutputSignals=h_R_valid
  Detect Rise Positive : simulink/Logic and Bit Operations/Detect Rise Positive  vinit=0  OutDataTypeStr=boolean
  Detect Rise Positive1 : simulink/Logic and Bit Operations/Detect Rise Positive  vinit=0  OutDataTypeStr=boolean
  pos_reset : Outport
  height_reset : Outport  Port=2
  wires:
  Detect Rise Positive/1 -> pos_reset/1
  Detect Rise Positive1/1 -> height_reset/1
  Bus Selector/1 -> Detect Rise Positive/1  "<xy_R_valid>"
  Bus Selector1/1 -> Detect Rise Positive1/1  "<h_R_valid>"
  Sensor_Valid/1 -> Bus Selector1/1, Bus Selector/1

== system INS/Data_Fusion/Translation_Filter/TF_Data_PreProcess/Transfer_Filter_Control/Position_Reference ==
  Sensor_Valid : Inport
  Translation_Data : Inport  Port=2
  Sensor_Meas : Inport  Port=3
  Bus_Constructor : Subsystem
  Bus_Select : Subsystem
  Height_Ref : Subsystem
  Position_Ref : Subsystem
  WGS84_Ref : Outport
  wires:
  Bus_Select/2(WGS84_position) -> Position_Ref/4(WGS84_position), Height_Ref/4(WGS84_position)
  Translation_Data/1 -> Height_Ref/1(Translation_Data), Position_Ref/1(Translation_Data)
  Sensor_Valid/1 -> Height_Ref/2(Sensor_Valid), Position_Ref/2(Sensor_Valid)
  Bus_Select/1(WGS84_derivatives) -> Height_Ref/3(WGS84_derivatives), Position_Ref/3(WGS84_derivatives)
  Position_Ref/1(WGS84_pos_ref) -> Bus_Constructor/1(WGS84_pos_ref)
  Position_Ref/2(WGS84_dpos_ref) -> Bus_Constructor/2(WGS84_dpos_ref)
  Height_Ref/1(WGS84_hgt_ref) -> Bus_Constructor/3(WGS84_hgt_ref)
  Height_Ref/2(WGS84_dhgt_ref) -> Bus_Constructor/4(WGS84_dhgt_ref)
  Bus_Constructor/1(WGS84_Ref) -> WGS84_Ref/1
  Sensor_Meas/1 -> Bus_Select/1(Sensor_Meas)

== system INS/Data_Fusion/Translation_Filter/TF_Data_PreProcess/Transfer_Filter_Control/Sensor_Valid ==
  Sensor_Enable : Inport
  Bus Creator : BusCreator  Inputs=4
  Horizon_Sensor_Valid : Subsystem
  Vertical_Sensor_Valid : Subsystem
  Sensor_Valid : Outport
  wires:
  Horizon_Sensor_Valid/1(lon_lat_valid) -> Bus Creator/1  "lon_lat_valid"
  Horizon_Sensor_Valid/2(xy_R_valid) -> Bus Creator/2  "xy_R_valid"
  Vertical_Sensor_Valid/1(altitude_valid) -> Bus Creator/3  "altitude_valid"
  Vertical_Sensor_Valid/2(h_R_valid) -> Bus Creator/4  "h_R_valid"
  Bus Creator/1 -> Sensor_Valid/1
  Sensor_Enable/1 -> Vertical_Sensor_Valid/1(Sensor_Enable), Horizon_Sensor_Valid/1(Sensor_Enable)

== system INS/Sensor_PreProcess/GPS_PreProcess/Status_Quality/GPS_Status/Ready ==
  valid : Inport
  Saturation : Saturate  UpperLimit=1e4  LowerLimit=0
  Sum : Sum  Inputs=|++  OutDataTypeStr=int32
  Unit Delay : UnitDelay  SampleTime=-1
  valid_samples : simulink/Logic and Bit Operations/Compare To Constant  relop=>=  const=1000  OutDataTypeStr=boolean
  ready : Outport
  wires:
  valid_samples/1 -> ready/1
  Sum/1 -> Saturation/1
  Unit Delay/1 -> valid_samples/1, Sum/2
  Saturation/1 -> Unit Delay/1
  valid/1 -> Sum/1

== system INS/Sensor_PreProcess/MAG_PreProcess/Mag_Data_Process/Mag_Quality_Estimate/Mag_Quality ==
  nominal_inc_deg : Inport
  mag_normalized_O : Inport  Port=2
  Inclination_Quality_Estimate : Subsystem
  Intensity_Quality_Estimate : Subsystem
  MinMax : MinMax  Inputs=2
  Second Order LPF : FMT_Model_Lib/Filter/Second Order LPF  fc=5  zeta=0.707
      settings: SourceProductName=FMT Toolbox
  mag_quality : Outport
  wires:
  Intensity_Quality_Estimate/1(intensity_quality) -> MinMax/2  "mag_int_quality"
  nominal_inc_deg/1 -> Inclination_Quality_Estimate/1(nominal_inc_deg)
  Inclination_Quality_Estimate/1(inclination_quality) -> MinMax/1  "mag_inc_quality"
  mag_normalized_O/1 -> Inclination_Quality_Estimate/2(mag_normalized_O), Intensity_Quality_Estimate/1(mag_normalized_O)
  MinMax/1 -> Second Order LPF/1
  Second Order LPF/1 -> mag_quality/1

== system INS/Sensor_PreProcess/MAG_PreProcess/Mag_Data_Process/WMM_Compensation/safe_divide ==
  u1 : Inport
  u2 : Inport  Port=2
  Constant1 : Constant  VectorParams1D=off  OutDataTypeStr=single
  Divide1 : Product  Inputs=*/
  MinMax : MinMax  Function=max  Inputs=2
  y : Outport
  wires:
  MinMax/1 -> Divide1/2
  Constant1/1 -> MinMax/1
  Divide1/1 -> y/1
  u2/1 -> MinMax/2
  u1/1 -> Divide1/1

== system INS/Data_Fusion/Rotation_Filter/AHRS/Correct/Attitude_Correction/Attitude_Correct ==
  Rotation_Data : Inport
  Sensor_Data : Inport  Port=2
  Acc_Correct : Subsystem
  Acc_Estimator : Subsystem
  att_corr_O : Outport
  wires:
  Acc_Estimator/3(acc_est_O_mPs2) -> Acc_Correct/3(acc_est_O_mPs2)  "acc_est_O_mPs2"
  Sensor_Data/1 -> Acc_Estimator/1(Sensor_Data)
  Rotation_Data/1 -> Acc_Estimator/2(Rotation_Data)
  Acc_Correct/1(att_correct) -> att_corr_O/1
  Acc_Estimator/1(acc_meas_valid) -> Acc_Correct/1(acc_meas_valid)  "acc_meas_valid"
  Acc_Estimator/2(acc_meas_O_mPs2) -> Acc_Correct/2(acc_meas_O_mPs2)  "acc_meas_O_mPs2"

== system INS/Data_Fusion/Rotation_Filter/AHRS/Correct/Attitude_Correction/Mag_Correct ==
  Rotation_Data : Inport
  Sensor_Data : Inport  Port=2
  standstill : Inport  Port=3
  Bus Selector1 : BusSelector  OutputSignals=Mag_Data.mag_norm_B,Mag_Data.mag_quality
  Bus Selector4 : BusSelector  OutputSignals=M_OB
  Logical Operator2 : Logic  AllPortsSameDT=off  OutDataTypeStr=boolean
  MX Product3 : Product  Inputs=3  RndMeth=Simplest
  MX Product4 : Product  Multiplication=Matrix(*)  RndMeth=Simplest
  Relay1 : Relay  OnSwitchValue=0.3  OffSwitchValue=0.2
  Selector2 : Selector  NumberOfDimensions=2  InputPortWidth=3  IndexOptions=Index vector (dialog),Index vector (dialog)  Indices=[3],[1 2 3]  OutputSizes=1,1
  Selector4 : Selector  NumberOfDimensions=2  InputPortWidth=3  IndexOptions=Index vector (dialog),Index vector (dialog)  Indices=[2],[1 2 3]  OutputSizes=1,1
  Subsystem : Subsystem  Commented=on
  Transpose2 : Math  Operator=transpose  SaturateOnIntegerOverflow=on
  mag_correct_gain : Gain  Gain=-INS_PARAM.MAG_CORR_GAIN  OutDataTypeStr=Inherit: Same as input
  mag_corr_O : Outport
  wires:
  Bus Selector4/1 -> Selector2/1, Selector4/1, Subsystem/1(M_OB)  "<M_OB>"
  Rotation_Data/1 -> Subsystem/3(Rotation_Data), Bus Selector4/1
  Bus Selector1/2 -> Relay1/1  "<mag_quality>"
  Bus Selector1/1 -> Subsystem/2(mag_B), MX Product4/2  "<mag_norm_B>"
  Sensor_Data/1 -> Bus Selector1/1
  MX Product3/1 -> mag_corr_O/1
  standstill/1 -> Logical Operator2/2
  Relay1/1 -> Logical Operator2/1
  Selector2/1 -> Transpose2/1
  mag_correct_gain/1 -> MX Product3/2
  MX Product4/1 -> mag_correct_gain/1  "my_O"
  Logical Operator2/1 -> MX Product3/3  "mag_enable"
  Transpose2/1 -> MX Product3/1  "Bz_O"
  Selector4/1 -> MX Product4/1

== system INS/Data_Fusion/Translation_Filter/CF/Bus_Constructor/Bus_Select/Bus_Select ==
  Horizontal_States : Inport
  Verticle_States : Inport  Port=2
  Mux : Mux  Inputs=2
  Mux1 : Mux  Inputs=2
  Mux2 : Mux  Inputs=2
  Selector : Selector  InputPortWidth=6  IndexOptions=Index vector (dialog)  Indices=[1 2]  OutputSizes=1
  Selector1 : Selector  InputPortWidth=3  IndexOptions=Index vector (dialog)  Indices=[1]  OutputSizes=1
  Selector2 : Selector  InputPortWidth=6  IndexOptions=Index vector (dialog)  Indices=[3 4]  OutputSizes=1
  Selector3 : Selector  InputPortWidth=3  IndexOptions=Index vector (dialog)  Indices=[2]  OutputSizes=1
  Selector4 : Selector  InputPortWidth=6  IndexOptions=Index vector (dialog)  Indices=[5 6]  OutputSizes=1
  Selector5 : Selector  InputPortWidth=3  IndexOptions=Index vector (dialog)  Indices=[3]  OutputSizes=1
  pos_R_m : Outport
  vel_O_mPs : Outport  Port=2
  ba_O_mPs2 : Outport  Port=3
  wires:
  Selector5/1 -> Mux2/2
  Horizontal_States/1 -> Selector4/1, Selector2/1, Selector/1
  Selector4/1 -> Mux2/1
  Selector2/1 -> Mux1/1
  Selector1/1 -> Mux/2
  Selector/1 -> Mux/1
  Selector3/1 -> Mux1/2
  Mux1/1 -> vel_O_mPs/1
  Verticle_States/1 -> Selector5/1, Selector3/1, Selector1/1
  Mux/1 -> pos_R_m/1
  Mux2/1 -> ba_O_mPs2/1

== system INS/Data_Fusion/Translation_Filter/CF/Bus_Constructor/Bus_Select/Local_Position ==
  xyh_R_m : Inport
  Demux : Demux  Outputs=3
  x_R_m : Outport
  y_R_m : Outport  Port=2
  h_R_m : Outport  Port=3
  wires:
  Demux/2 -> y_R_m/1
  Demux/1 -> x_R_m/1
  Demux/3 -> h_R_m/1
  xyh_R_m/1 -> Demux/1

== system INS/Data_Fusion/Translation_Filter/CF/Bus_Constructor/Bus_Select/Velocity ==
  vel_O_mPs : Inport
  Demux : Demux  Outputs=3
  vn_mPs : Outport
  ve_mPs : Outport  Port=2
  vd_mPs : Outport  Port=3
  wires:
  Demux/3 -> vd_mPs/1
  Demux/1 -> vn_mPs/1
  Demux/2 -> ve_mPs/1
  vel_O_mPs/1 -> Demux/1

== system INS/Data_Fusion/Translation_Filter/CF/Bus_Constructor/Bus_Select/WGS84_Position ==
  TF_Data : Inport
  xyh_R_m : Inport  Port=2
  Bus Selector2 : BusSelector  OutputSignals=Sensor_Status.GPS_Status.gps_vaid
  Data Type Conversion2 : DataTypeConversion  OutDataTypeStr=double
  Demux2 : Demux  Outputs=3
  Multiply : Product
  WGS84_Position : Subsystem
  lat_rad : Outport
  lon_rad : Outport  Port=2
  h_m : Outport  Port=3
  wires:
  WGS84_Position/1(WGS84_pos) -> Multiply/2
  TF_Data/1 -> Bus Selector2/1, WGS84_Position/2(TF_Data)
  Bus Selector2/1 -> Data Type Conversion2/1  "<gps_vaid>"
  Data Type Conversion2/1 -> Multiply/1
  Multiply/1 -> Demux2/1
  xyh_R_m/1 -> WGS84_Position/1(xyh_R_m)
  Demux2/1 -> lat_rad/1  "lat_rad"
  Demux2/2 -> lon_rad/1  "lon_rad"
  Demux2/3 -> h_m/1  "h_m"

== system INS/Data_Fusion/Translation_Filter/CF/Horizontal_Filter/Correct/GPS_Correct ==
  TF_Data : Inport
  X_Predict : Inport  Port=2
  Enable : EnablePort  StatesWhenEnabling=reset
  Bus Selector : BusSelector  OutputSignals=TF_Control.pos_reset
  Bus Selector1 : BusSelector  OutputSignals=Sensor_Meas.GPS_Meas.timestamp_ms
  Detect Change : simulink/Logic and Bit Operations/Detect Change  vinit=0  OutDataTypeStr=boolean
  Error_Integrate : Subsystem
  Error_Scaling : Subsystem
  Estimate_State : Subsystem
  Logical Operator : Logic  Operator=OR  AllPortsSameDT=off  OutDataTypeStr=boolean
  Measurement : Subsystem
  Sum : Sum  Inputs=|-+
  Sum1 : Sum  Inputs=++|
  X_Next : Outport
  wires:
  Estimate_State/1(HX) -> Sum/1  "gps_state_hor_O"
  Measurement/1(Z) -> Sum/2  "gps_meas_hor_O"
  TF_Data/1 -> Bus Selector/1, Measurement/2(TF_Data), Bus Selector1/1
  Sum/1 -> Error_Scaling/1(err_in)  "gps_error_hor_O"
  Bus Selector1/1 -> Detect Change/1  "<timestamp_ms>"
  Error_Integrate/1(corr) -> Sum1/2
  Sum1/1 -> X_Next/1
  X_Predict/1 -> Estimate_State/1(X), Measurement/1(X), Sum1/1
  Bus Selector/1 -> Estimate_State/2(reset)  "<pos_reset>"
  Logical Operator/1 -> Error_Integrate/2(update)
  Detect Change/1 -> Logical Operator/2
  Measurement/2(bias_update) -> Logical Operator/1
  Error_Scaling/1(err_out) -> Error_Integrate/1(error)

== system INS/Data_Fusion/Translation_Filter/CF/Horizontal_Filter/Predict/Propagate ==
  X_prio : Inport
  TF_Data : Inport  Port=2
  Bus Selector : BusSelector  OutputSignals=TF_Control.pos_reset
  Delay : Delay  DelayLength=1
  States_Init : Subsystem
  Switch : Switch  Criteria=u2 > Threshold
  X : Outport
  wires:
  Delay/1 -> Switch/3
  States_Init/1(X_0) -> Switch/1
  Switch/1 -> X/1
  Bus Selector/1 -> Switch/2  "<pos_reset>"
  TF_Data/1 -> Bus Selector/1, States_Init/1(TF_Data)
  X_prio/1 -> Delay/1

== system INS/Data_Fusion/Translation_Filter/CF/Horizontal_Filter/Predict/Update ==
  X_Prio : Inport
  Rotation_Data : Inport  Port=2
  Add : Sum  Inputs=-+
  Bus Selector2 : BusSelector  OutputSignals=M_OB,acc_B_mPs2
  Constant : Constant  Value=[0;0]  OutDataTypeStr=single
  Gain : Gain  Gain=INS_CONST.dt  OutDataTypeStr=Inherit: Same as input
  Multiply : Product  Multiplication=Matrix(*)
  Mux : Mux  Inputs=3
  Reshape : Reshape  OutputDimensionality=Customize  OutputDimensions=[6,1]
  Selector : Selector  InputPortWidth=3  IndexOptions=Index vector (dialog)  Indices=[1 2]  OutputSizes=1
  Selector1 : Selector  InputPortWidth=6  IndexOptions=Index vector (dialog)  Indices=[3 4]  OutputSizes=1
  Selector2 : Selector  InputPortWidth=6  IndexOptions=Index vector (dialog)  Indices=[5 6]  OutputSizes=1
  Sum : Sum  Inputs=++|
  X_Predict : Outport
  wires:
  Rotation_Data/1 -> Bus Selector2/1
  Bus Selector2/1 -> Multiply/1  "<M_OB>"
  Multiply/1 -> Selector/1  "acc_O"
  Bus Selector2/2 -> Multiply/2  "<acc_B_mPs2>"
  X_Prio/1 -> Selector1/1, Sum/1, Selector2/1
  Selector/1 -> Add/2
  Selector1/1 -> Mux/1
  Constant/1 -> Mux/3
  Mux/1 -> Reshape/1
  Reshape/1 -> Gain/1
  Sum/1 -> X_Predict/1
  Gain/1 -> Sum/2
  Add/1 -> Mux/2
  Selector2/1 -> Add/1

== system INS/Data_Fusion/Translation_Filter/CF/Verticle_Filter/Correct/Baro_Correct ==
  X_Predict : Inport
  TF_Data : Inport  Port=2
  Baro_Correct : Subsystem
  Bus Selector : BusSelector  OutputSignals=Sensor_Enable.vert_select.baro_enable
  Switch : Switch  Criteria=u2 > Threshold
  X_Next : Outport
  wires:
  Switch/1 -> X_Next/1
  Bus Selector/1 -> Baro_Correct/Enable, Switch/2  "<baro_enable>"
  TF_Data/1 -> Baro_Correct/1(TF_Data), Bus Selector/1
  Baro_Correct/1(X_Next) -> Switch/1
  X_Predict/1 -> Baro_Correct/2(X_Predict), Switch/3

== system INS/Data_Fusion/Translation_Filter/CF/Verticle_Filter/Correct/GPS_Correct ==
  X_Predict : Inport
  TF_Data : Inport  Port=2
  Bus Selector : BusSelector  OutputSignals=Sensor_Enable.vert_select.gps_enable
  GPS_Correct : Subsystem
  Switch : Switch  Criteria=u2 > Threshold
  X_Next : Outport
  wires:
  Switch/1 -> X_Next/1
  Bus Selector/1 -> GPS_Correct/Enable, Switch/2  "<gps_enable>"
  TF_Data/1 -> GPS_Correct/1(TF_Data), Bus Selector/1
  GPS_Correct/1(X_Next) -> Switch/1
  X_Predict/1 -> GPS_Correct/2(X_Predict), Switch/3

== system INS/Data_Fusion/Translation_Filter/CF/Verticle_Filter/Predict/Propagate ==
  X_Prio : Inport
  TF_Data : Inport  Port=2
  Bus Selector : BusSelector  OutputSignals=TF_Control.height_reset
  Delay : Delay  DelayLength=1
  States_Init : Subsystem
  Switch : Switch  Criteria=u2 > Threshold
  X : Outport
  wires:
  X_Prio/1 -> Delay/1
  TF_Data/1 -> States_Init/1(TF_Data), Bus Selector/1
  Bus Selector/1 -> Switch/2  "<height_reset>"
  Switch/1 -> X/1
  States_Init/1(X_0) -> Switch/1
  Delay/1 -> Switch/3
